simulink model "mouthDet_template_R2010b"  (Simulink 7.2)
settings: Solver=FixedStepDiscrete  StartTime=0.0  StopTime=inf  RelTol=1e-3
undefined symbols (not defined in the file or in its folder): gray, jet, Rec, SDTV, strel
libraries: vipsnks x5, vipmorphops x2, simulink x2, vipstatistics x1, vipconversions x1, dspsrcs4 x1, vipanalysis x1
settings Model: Creator=Jaromir  LastModifiedBy=virtual
settings DebuggingCC: StrictBusMsg=ErrorLevel1

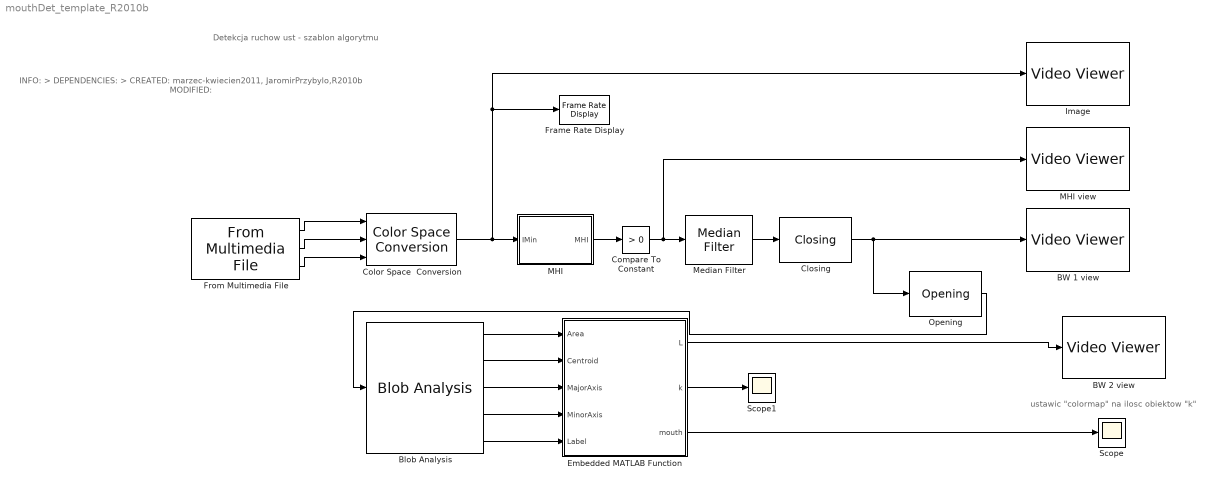
== system mouthDet_template_R2010b ==
  note: Detekcja ruchow ust - szablon algorytmu
  note: INFO:
      |  >
      | DEPENDENCIES:
      |  >
      | CREATED: marzec-kwiecien2011, JaromirPrzybylo,R2010b
      | MODIFIED:
  note: ustawic "colormap" na ilosc obiektow "k"
  BW 1 view : vipsnks/Video Viewer  DialogController=vipDDGCreate  DialogControllerArgs=DataTag1  inputType=Obsolete7b  imagePorts=One multidimensional signal  useColorMap=off  colormapValue=gray(256)  specRange=on  minInputVal=0  maxInputVal=1  FigPos=[735 579 640 480]  AxisZoom=on  trueSizedOnce=on
  BW 2 view : vipsnks/Video Viewer  DialogController=vipDDGCreate  DialogControllerArgs=DataTag3  inputType=Obsolete7b  imagePorts=One multidimensional signal  useColorMap=on  colormapValue=jet(11)  specRange=on  minInputVal=0  maxInputVal=10  FigPos=[1 854 640 480]  AxisZoom=on  trueSizedOnce=on
  Blob Analysis : vipstatistics/Blob Analysis  Tag=vipblks_row_conv  DialogController=vipDDGCreate  DialogControllerArgs=DataTag4  area=on  centroid=on  bBox=off  majorAxis=on  minorAxis=on  angle=off  eccentricity=off  equivDiameterSq=off  extent=off  perimeter=off  maxBlobs=250  warnIfNumBlobsExceeded=on  isCount=off  useMinArea=off  minArea=0  useMaxArea=off  maxArea=intmax('uint32')  excludeBorderBlob=off  outDT=double  isOutVarDim=off  isFill=on  fillValues=-1  conn=8  isLabel=on  outputMode=Binary point scaling  outputWordLength=32  outputFracLength=16  firstCoeffMode=Binary point scaling  firstCoeffWordLength=16  firstCoeffFracLength=14  secondCoeffMode=Binary point scaling  secondCoeffWordLength=32  secondCoeffFracLength=16  accumMode=Binary point scaling  accumWordLength=32  accumFracLength=0  prodOutputMode=Binary point scaling  prodOutputWordLength=32  prodOutputFracLength=16  roundingMode=Floor  overflowMode=off
  Closing : vipmorphops/Closing  nhoodsrc=Specify via dialog  strel=strel('disk',3)
  Color Space  Conversion : vipconversions/Color Space  Conversion  conversion=Obsolete  conversionActive=R'G'B' to intensity  wp_str=D65  rec=Rec. 601 (SDTV)  sys=1125/60/2:1  imagePorts=Separate color signals
  Compare To Constant : simulink/Logic and Bit Operations/Compare To Constant  SystemSampleTime=-1  relop=>  const=0  LogicOutDataTypeMode=boolean
  Embedded MATLAB Function : Stateflow chart  TreatAsAtomicUnit=on
  Frame Rate Display : vipsnks/Frame Rate Display  DialogController=vipDDGCreate  DialogControllerArgs=DataTag5  UpdateRate=10
  From Multimedia File : dspsrcs4/From Multimedia File  DialogController=dspDDGCreate  DialogControllerArgs=DataTag6  inputFilename=Y:\Studia\Informatyka Stosowana\III rok\Interfejsy multimodalne\labolatorium\projekt\Multimodal\test_movie.avi  loop=on  numPlays=inf  outputStreams=Video only  videoDataType=uint8  audioDataType=int16  inheritSampleTime=off  userDefinedSampleTime=1  noAudioOutput=off  isIntensityVideo=off  colorVideoFormat=Separate color signals  outputEOF=off  dataOrg=Column-major
  Image : vipsnks/Video Viewer  DialogController=vipDDGCreate  DialogControllerArgs=DataTag8  inputType=Obsolete7b  imagePorts=One multidimensional signal  useColorMap=off  colormapValue=jet(256)  specRange=off  minInputVal=0  maxInputVal=255  FigPos=[1 579 640 480]  AxisZoom=on  trueSizedOnce=on
  MHI : Subsystem  mask{tres=9, Tau=5}
      mask prompts: tres "Motion treshold"; Tau "Tau parameter"
  MHI view : vipsnks/Video Viewer  DialogController=vipDDGCreate  DialogControllerArgs=DataTag10  inputType=Obsolete7b  imagePorts=One multidimensional signal  useColorMap=off  colormapValue=gray(256)  specRange=on  minInputVal=0  maxInputVal=1  FigPos=[318 579 640 480]  AxisZoom=on  trueSizedOnce=on
  Median Filter : vipanalysis/Median Filter  DialogController=vipDDGCreate  DialogControllerArgs=DataTag11  nghbood=[3 3]  outSize=Same as input port I  padType=Constant  padSrc=Specify via dialog  padVal=0  roundingMode=Floor  overflowMode=off
  Opening : vipmorphops/Opening  nhoodsrc=Specify via dialog  strel=strel('disk',3)
  Scope : Scope
  Scope1 : Scope
  wires:
  From Multimedia File/1 -> Color Space  Conversion/1
  From Multimedia File/2 -> Color Space  Conversion/2
  From Multimedia File/3 -> Color Space  Conversion/3
  Color Space  Conversion/1 -> MHI/1(IMin), Image/1, Frame Rate Display/1
  MHI/1(MHI) -> Compare To Constant/1
  Compare To Constant/1 -> Median Filter/1, MHI view/1
  Median Filter/1 -> Closing/1
  Closing/1 -> BW 1 view/1, Opening/1
  Blob Analysis/1 -> Embedded MATLAB Function/1(Area)
  Blob Analysis/2 -> Embedded MATLAB Function/2(Centroid)
  Blob Analysis/3 -> Embedded MATLAB Function/3(MajorAxis)
  Blob Analysis/4 -> Embedded MATLAB Function/4(MinorAxis)
  Blob Analysis/5 -> Embedded MATLAB Function/5(Label)
  Embedded MATLAB Function/1(L) -> BW 2 view/1
  Embedded MATLAB Function/3(mouth) -> Scope/1
  Embedded MATLAB Function/2(k) -> Scope1/1
  Opening/1 -> Blob Analysis/1

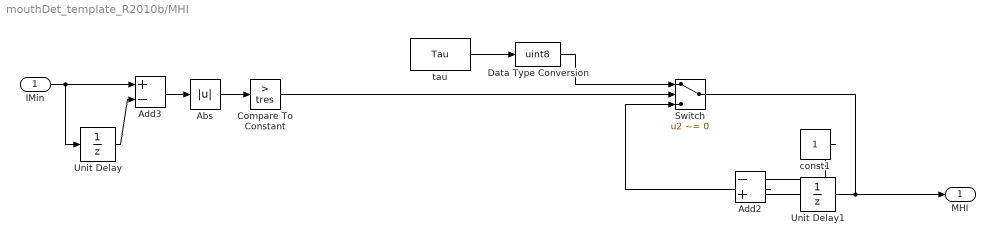
== system mouthDet_template_R2010b/MHI ==
  IMin : Inport
  Abs : Abs  OutDataTypeMode=Specify via dialog  OutDataType=fixdt(0,9,0)  OutDataTypeStr=fixdt(0,9,0)
  Add2 : Sum  Inputs=-+  OutDataTypeMode=uint8  OutDataTypeStr=uint8  SaturateOnIntegerOverflow=on
  Add3 : Sum  Inputs=+-  AccumDataTypeStr=fixdt(1,9,0)  OutDataTypeMode=Specify via dialog  OutDataType=fixdt(1,9,0)  OutDataTypeStr=fixdt(1,9,0)
  Compare To Constant : simulink/Logic and Bit Operations/Compare To Constant  SystemSampleTime=-1  relop=>  const=tres  LogicOutDataTypeMode=uint8  ZeroCross=off
  Data Type Conversion : DataTypeConversion  OutDataTypeMode=uint8  OutDataTypeStr=uint8
  Switch : Switch  Criteria=u2 ~= 0
  Unit Delay : UnitDelay  SampleTime=-1
  Unit Delay1 : UnitDelay  SampleTime=-1
  const1 : Constant  OutDataTypeMode=uint8  OutDataTypeStr=uint8
  tau : Constant  Value=Tau
  MHI : Outport
  wires:
  Abs/1 -> Compare To Constant/1
  tau/1 -> Data Type Conversion/1
  Switch/1 -> Unit Delay1/1, MHI/1
  Unit Delay1/1 -> Add2/2
  const1/1 -> Add2/1
  Add2/1 -> Switch/3
  IMin/1 -> Unit Delay/1, Add3/1
  Add3/1 -> Abs/1
  Unit Delay/1 -> Add3/2
  Compare To Constant/1 -> Switch/2
  Data Type Conversion/1 -> Switch/1

== matlab function Embedded MATLAB Function ==
  data: Area input double; L output double; k output double; Centroid input double; MajorAxis input double; MinorAxis input double; Label input double; mouth output double
function [L,k,mouth]  = analiza_szablon(Area, Centroid, MajorAxis, MinorAxis, Label)
%#eml
% Analiza i detekcja mrugniec
% INPUTS:
% > Area, Centroid, MajorAxis, MinorAxis, Label
%    dane z bloku "Blob analysis"
% OUTPUTS:
% > L     - obraz indeksowany po analizie
% > k     - ilosc obiektow po analizie
% > mouth - sygnal [0,1] informujacy o fakcie detekcji ruchu ust
% COMMENTS:
% - uzupelnic w ramach miniprojektu
%

[m,n]=size(Label);
ilobj=length(Area);

L=zeros(m,n,'uint8');
mouth=0;

% Analiza
i=1;k=1;
for i=1:ilobj
    % Sprawdzenie wielkosci obiektow
    if Area(i) > 200 && Area(i) < (m*n*0.5)
        L=L + uint8(Label==i)*k;
        k=k+1;
    end
end
